simulink model "controller_dist_def_controller"  (R2018b)
settings: Solver=VariableStepAuto  StartTime=0.0  StopTime=30  MaxStep=1e-3  RelTol=1e-3
InitFcn:
  | % NOTE: If using VoltPAQ-X1, make sure both Gain switches are set to 3.
  | K_AMP = 3;
  | % Maximum Output Voltage (V): YAW limited to 15 V. PITCH limited to 24 V.
  | VMAX_AMP_P = 24;
  | VMAX_AMP_Y = 15;
  | % Initial Angle of Pitch (rad)
  | theta_0 = -40.5*pi/180;
  | 
  | g = 9.81;
  | 
  | % Pitch and Yaw Motor Armature Resistance (Ohm)
  | R_m_p = 0.83;
  | R_m_y = 1.60;
  | 
  | % Pitch and Yaw Motor Current-Torque Constant (N.m/A)
  | K_t_p = 0.0182;
  | K_t_y = 0.0109;
  | 
  | % Pitch and Yaw Motor Voltage-Torque Constant (N.m/V)
  | K_yp = K_t_p / R_m_p;
  | K_py = K_t_y / R_m_y;
  | 
  | % Pitch and Yaw Viscous Damping Constant (N.m.s/rad)
  | B_p = 0.8;  % tuned while running simulation and experiment in parallel
  | B_y = 0.318; % identified as described in manual
  | 
  | % Mass of the Helicopter (kg)
  | m_heli = 1.3872;
  | 
  | % Mass of the Helicopter with Yoke (kg)
  | m_heli_case = 1.421;
  | 
  | % Distance from Pitch Pivot to Pitch/Front Motor and Yaw/Back Motor(m)
  | r_p = 7.75*0.0254;
  | r_y = (6+5/8)*0.0254;
  | 
  | % Pitch and Yaw Propeller Force-Thrust Constant found Experimentally (N/V)
  | K_f_p = 5*0.2074;
  | K_f_y = 3*0.1426;
  | 
  | % Pitch and Yaw Propeller Torque-Thrust Constant found Experimentally (N.m/V)
  | K_pp = K_f_p * r_p;
  | K_yy = K_f_y * r_y;
  | 
  | % Mass of Pitch/Front Motor and Yaw/Back Motor (kg)
  | m_motor_p = 0.292;
  | m_motor_y = 0.128;
  | 
  | % Mass of Pitch/Front and Yaw/Back Guard + Propeller(kg)
  | m_shield = 0.143 + 0.024;
  | 
  | % Total Mass of Pitch and Yaw Motor/Shield Assemblies (kg)
  | m_props = ( m_motor_p + m_motor_y + 2 * m_shield );
  | 
  | % Mass of Helicopter Body moving about Pitch Axis (kg)
  | m_body_p = m_heli - m_props;
  | 
  | % Mass of Helicopter Body moving about Yaw Axis (kg)
  | m_body_y = m_heli_case - m_props;
  | 
  | % Mass of Metal Shaft Moving about Yaw Axis (kg)
  | m_shaft = 0.151;
  | 
  | % Total Length of Helicopter Body (m)
  | L_body = 19*0.0254;
  | 
  | % Helicopter Center of Mass from Pivot along Pitch Axis (m)
  | l_cm = ( (m_motor_p + m_shield ) * r_p +  (m_motor_y + m_shield ) * r_y ) / ( m_props ) ;
  | 
  | % Length of Metal Shaft Moving about Yaw Axis through slip ring (m)
  | L_shaft = 11 * 0.0254;
  | 
  | % Pitch and Yaw Motor Rotor Moment of Inertia (kg.m^2)
  | J_m_p = 1.91e-6; %1.7070e-5;
  | J_m_y = 1.374e-4; %1.4471e-5;
  | 
  | % Moment of Inertia of Helicopter Body about its CM (kg.m^2)
  | J_body_p = m_body_p * L_body^2 / 12;
  | J_body_y = m_body_y * L_body^2 / 12;
  | 
  | % Moment of Inertia of Metal Shaft about Yaw Axis (kg.m^2)
  | J_shaft = m_shaft * L_shaft^2 / 3; %;0.0851;
  | 
  | % Moment of Inertia of Pitch Motor + Guard Assembly about Pivot (kg.m^2)
  | J_p = ( m_motor_p + m_shield ) * r_p^2;
  | 
  | % Moment of Inertia of Yaw Motor + Guard Assembly about Pivot (kg.m^2)
  | J_y = ( m_motor_y + m_shield ) * r_y^2;
  | 
  | % Equivalent Moment of Inertia about Pitch and Yaw Axis (kg.m^2)
  | J_eq_p = J_m_p + J_body_p + J_p + J_y;
  | J_eq_y = J_m_y + J_body_y + J_p + J_y + J_shaft;
  | 
  | 
  | %BESSEL wn=4
  | Kbes=[     68.5119  -25.1203    5.3421   -3.6881
  |    63.1652  188.4894    0.7783   19.4789];
  | 
  | xd=-20;
settings Model: Creator=rezan  LastModifiedBy=rezan
settings DataIOCC: ReturnWorkspaceOutputs=on
settings DebuggingCC: UnconnectedInputMsg=none  UnconnectedOutputMsg=none  UnconnectedLineMsg=none  SFMachineParentedDataDiag=error

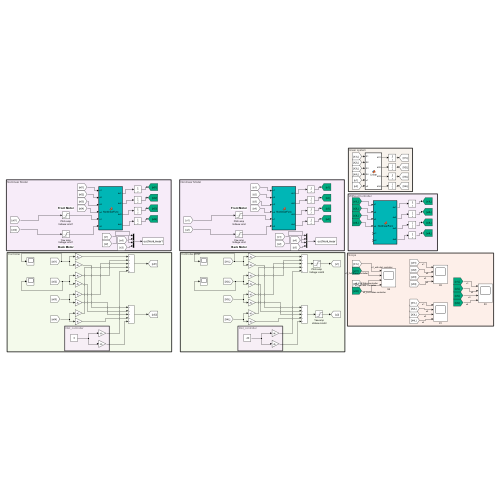
[thumbnail: Simulink's stored preview of the top-level diagram]
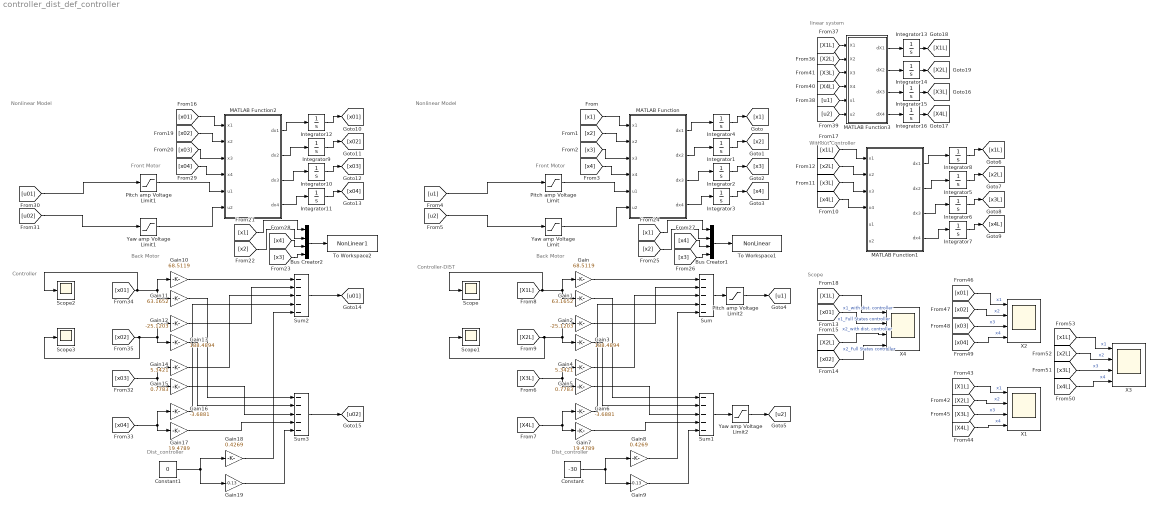
== system controller_dist_def_controller ==
  note: Dist_controller
  note: Controller-DIST
  note: Scope
  note: Nonlinear Model
  note: Front Motor
  note: Back Motor
  note: Without Controller
  note: Dist_controller
  note: Controller
  note: Nonlinear Model
  note: Front Motor
  note: Back Motor
  note: linear system
  Bus Creator1 : BusCreator  Inputs=4
  Bus Creator2 : BusCreator  Inputs=4
  Constant : Constant  Value=-30
  Constant1 : Constant  Value=0
  Gain : Gain  Gain=68.5119
  Gain1 : Gain  Gain=63.1652
  Gain10 : Gain  Gain=68.5119
  Gain11 : Gain  Gain=63.1652
  Gain12 : Gain  Gain=-25.1203
  Gain13 : Gain  Gain=188.4894
  Gain14 : Gain  Gain=5.3421
  Gain15 : Gain  Gain=0.7783
  Gain16 : Gain  Gain=-3.6881
  Gain17 : Gain  Gain=19.4789
  Gain18 : Gain  Gain=0.4269
  Gain19 : Gain  Gain=-0.13
  Gain2 : Gain  Gain=-25.1203
  Gain3 : Gain  Gain=188.4894
  Gain4 : Gain  Gain=5.3421
  Gain5 : Gain  Gain=0.7783
  Gain6 : Gain  Gain=-3.6881
  Gain7 : Gain  Gain=19.4789
  Gain8 : Gain  Gain=0.4269
  Gain9 : Gain  Gain=-0.13
  Integrator{1..3,5,7,9,11,14,16} (9 alike) : Integrator
  Integrator10 : Integrator  InitialCondition=5
  Integrator{4,8,12..13} (4 alike) : Integrator  UpperSaturationLimit=40.5*pi/180  LowerSaturationLimit=-40.5*pi/180
  Integrator15 : Integrator  InitialCondition=5
  Integrator6 : Integrator  InitialCondition=5
  MATLAB Function : MATLAB Function  TreatAsAtomicUnit=on
  MATLAB Function1 : MATLAB Function  TreatAsAtomicUnit=on
  MATLAB Function2 : MATLAB Function  TreatAsAtomicUnit=on
  MATLAB Function3 : MATLAB Function  TreatAsAtomicUnit=on
  Pitch amp Voltage Limit : Saturate  UpperLimit=VMAX_AMP_P  LowerLimit=- VMAX_AMP_P
  Pitch amp Voltage Limit1 : Saturate  UpperLimit=VMAX_AMP_P  LowerLimit=- VMAX_AMP_P
  Pitch amp Voltage Limit2 : Saturate  UpperLimit=VMAX_AMP_P  LowerLimit=- VMAX_AMP_P
  Scope{,1..3} (4 alike) : Scope
  Sum{,1..3} (4 alike) : Sum  Inputs=-----
  To Workspace1 : ToWorkspace  VariableName=NonLinear  SampleTime=-1
  To Workspace2 : ToWorkspace  VariableName=NonLinear1  SampleTime=-1
  X{1..4} (4 alike) : Scope  NumInputPorts=4
  Yaw amp Voltage Limit : Saturate  UpperLimit=VMAX_AMP_Y  LowerLimit=- VMAX_AMP_Y
  Yaw amp Voltage Limit1 : Saturate  UpperLimit=VMAX_AMP_Y  LowerLimit=- VMAX_AMP_Y
  Yaw amp Voltage Limit2 : Saturate  UpperLimit=VMAX_AMP_Y  LowerLimit=- VMAX_AMP_Y
  wires:
  [x4] -> MATLAB Function/4(x4)
  [x2] -> MATLAB Function/2(x2)
  Integrator1/1 -> [x2]
  [u1] -> Pitch amp Voltage Limit/1
  [x1] -> MATLAB Function/1(x1)
  [u2] -> Yaw amp Voltage Limit/1
  MATLAB Function/1(dx1) -> Integrator4/1
  MATLAB Function/3(dx3) -> Integrator2/1
  MATLAB Function/2(dx2) -> Integrator1/1
  [x2] -> Bus Creator1/2
  [x4] -> Bus Creator1/3
  [x3] -> Bus Creator1/4
  Bus Creator1/1 -> To Workspace1/1
  Yaw amp Voltage Limit/1 -> MATLAB Function/6(u2)
  [x1] -> Bus Creator1/1
  Integrator3/1 -> [x4]
  Integrator4/1 -> [x1]
  MATLAB Function/4(dx4) -> Integrator3/1
  [x3] -> MATLAB Function/3(x3)
  Integrator2/1 -> [x3]
  Pitch amp Voltage Limit/1 -> MATLAB Function/5(u1)
  [X1L] -> Scope/1, Gain1/1, Gain/1
  [X4L] -> Gain7/1, Gain6/1
  [X3L] -> Gain4/1, Gain5/1
  Gain/1 -> Sum/1
  Gain2/1 -> Sum/2
  Gain4/1 -> Sum/3
  Gain6/1 -> Sum/4
  Gain3/1 -> Sum1/2
  Gain1/1 -> Sum1/1
  Gain5/1 -> Sum1/3
  Gain7/1 -> Sum1/4
  Sum/1 -> Pitch amp Voltage Limit2/1
  Sum1/1 -> Yaw amp Voltage Limit2/1
  Constant/1 -> Gain9/1, Gain8/1
  Gain8/1 -> Sum/5
  Gain9/1 -> Sum1/5
  [X2L] -> Scope1/1, Gain2/1, Gain3/1
  Integrator6/1 -> [x3L]
  Integrator8/1 -> [x1L]
  MATLAB Function1/4(dx4) -> Integrator7/1
  Integrator7/1 -> [x4L]
  [x3L] -> MATLAB Function1/3(x3)
  [x1L] -> MATLAB Function1/1(x1)
  MATLAB Function1/1(dx1) -> Integrator8/1
  MATLAB Function1/2(dx2) -> Integrator5/1
  [x2L] -> MATLAB Function1/2(x2)
  Integrator5/1 -> [x2L]
  MATLAB Function1/3(dx3) -> Integrator6/1
  [x4L] -> MATLAB Function1/4(x4)
  [X1L] -> X4/1  "x1_with dist. controller"
  [x01] -> X4/2  "x1_Full States controller"
  [X2L] -> X4/3  "x2_with dist. controller"
  [x02] -> X4/4  "x2_Full States controller"
  [x02] -> Gain13/1, Gain12/1, Scope3/1
  Gain19/1 -> Sum3/5
  Gain18/1 -> Sum2/5
  Constant1/1 -> Gain18/1, Gain19/1
  Sum3/1 -> [u02]
  Sum2/1 -> [u01]
  Gain17/1 -> Sum3/4
  Gain15/1 -> Sum3/3
  Gain11/1 -> Sum3/1
  Gain13/1 -> Sum3/2
  Gain16/1 -> Sum2/4
  Gain14/1 -> Sum2/3
  Gain12/1 -> Sum2/2
  Gain10/1 -> Sum2/1
  [x03] -> Gain15/1, Gain14/1
  [x04] -> Gain16/1, Gain17/1
  [x01] -> Gain10/1, Gain11/1, Scope2/1
  Pitch amp Voltage Limit1/1 -> MATLAB Function2/5(u1)
  Integrator10/1 -> [x03]
  [x03] -> MATLAB Function2/3(x3)
  MATLAB Function2/4(dx4) -> Integrator11/1
  Integrator12/1 -> [x01]
  Integrator11/1 -> [x04]
  [x1] -> Bus Creator2/1
  Yaw amp Voltage Limit1/1 -> MATLAB Function2/6(u2)
  Bus Creator2/1 -> To Workspace2/1
  [x3] -> Bus Creator2/4
  [x4] -> Bus Creator2/3
  [x2] -> Bus Creator2/2
  MATLAB Function2/2(dx2) -> Integrator9/1
  MATLAB Function2/3(dx3) -> Integrator10/1
  MATLAB Function2/1(dx1) -> Integrator12/1
  [u02] -> Yaw amp Voltage Limit1/1
  [x01] -> MATLAB Function2/1(x1)
  [u01] -> Pitch amp Voltage Limit1/1
  Integrator9/1 -> [x02]
  [x02] -> MATLAB Function2/2(x2)
  [x04] -> MATLAB Function2/4(x4)
  Integrator15/1 -> [X3L]
  [X4L] -> MATLAB Function3/4(X4)
  [X3L] -> MATLAB Function3/3(X3)
  MATLAB Function3/3(dX3) -> Integrator15/1
  MATLAB Function3/1(dX1) -> Integrator13/1
  MATLAB Function3/4(dX4) -> Integrator16/1
  Integrator13/1 -> [X1L]
  Integrator16/1 -> [X4L]
  MATLAB Function3/2(dX2) -> Integrator14/1
  [u1] -> MATLAB Function3/5(u1)
  [u2] -> MATLAB Function3/6(u2)
  [X2L] -> MATLAB Function3/2(X2)
  Integrator14/1 -> [X2L]
  [X1L] -> MATLAB Function3/1(X1)
  Pitch amp Voltage Limit2/1 -> [u1]
  Yaw amp Voltage Limit2/1 -> [u2]
  [X1L] -> X1/1  "x1"
  [X2L] -> X1/2  "x2"
  [X3L] -> X1/3  "x3"
  [X4L] -> X1/4  "x4"
  [x01] -> X2/1  "x1"
  [x02] -> X2/2  "x2"
  [x03] -> X2/3  "x3"
  [x04] -> X2/4  "x4"
  [x4L] -> X3/4  "x4"
  [x3L] -> X3/3  "x3"
  [x2L] -> X3/2  "x2"
  [x1L] -> X3/1  "x1"

== matlab function controller_dist_def_controller/MATLAB Function1 ==
  data: x1 input; x2 input; x3 input; x4 input; u1 input; dx1 output; u2 input; dx2 output; dx3 output; dx4 output
function [dx1,dx2,dx3,dx4]= NonlinearFunc(x1,x2,x3,x4,u1,u2)
%% Initial Conditions
% Gravitational Constant (m/s^2)
g = 9.81;

% Pitch and Yaw Motor Armature Resistance (Ohm)
R_m_p = 0.83;
R_m_y = 1.60;

% Pitch and Yaw Motor Current-Torque Constant (N.m/A)
K_t_p = 0.0182;
K_t_y = 0.0109;

% Pitch and Yaw Motor Voltage-Torque Constant (N.m/V)
K_yp = K_t_p / R_m_p;
K_py = K_t_y / R_m_y;

% Pitch and Yaw Viscous Damping Constant (N.m.s/rad)
B_p = 0.8;  % tuned while running simulation and experiment in parallel
B_y = 0.318; % identified as described in manual 

% Mass of the Helicopter (kg)
m_heli = 1.3872;

% Mass of the Helicopter with Yoke (kg)
m_heli_case = 1.421;

% Distance from Pitch Pivot to Pitch/Front Motor and Yaw/Back Motor(m)
r_p = 7.75*0.0254;
r_y = (6+5/8)*0.0254;

% Pitch and Yaw Propeller Force-Thrust Constant found Experimentally (N/V)
K_f_p = 5*0.2074;
K_f_y = 3*0.1426;

% Pitch and Yaw Propeller Torque-Thrust Constant found Experimentally (N.m/V)
K_pp = K_f_p * r_p;
K_yy = K_f_y * r_y;

% Mass of Pitch/Front Motor and Yaw/Back Motor (kg)
m_motor_p = 0.292;
m_motor_y = 0.128;

% Mass of Pitch/Front and Yaw/Back Guard + Propeller(kg)
m_shield = 0.143 + 0.024;

% Total Mass of Pitch and Yaw Motor/Shield Assemblies (kg)
m_props = ( m_motor_p + m_motor_y + 2 * m_shield );

% Mass of Helicopter Body moving about Pitch Axis (kg)
m_body_p = m_heli - m_props; 

% Mass of Helicopter Body moving about Yaw Axis (kg)
m_body_y = m_heli_case - m_props; 

% Mass of Metal Shaft Moving about Yaw Axis (kg)
m_shaft = 0.151;

% Total Length of Helicopter Body (m)
L_body = 19*0.0254;

% Helicopter Center of Mass from Pivot along Pitch Axis (m)
l_cm = ( (m_motor_p + m_shield ) * r_p +  (m_motor_y + m_shield ) * r_y ) / ( m_props ) ;

% Length of Metal Shaft Moving about Yaw Axis through slip ring (m)
L_shaft = 11 * 0.0254;

% Pitch and Yaw Motor Rotor Moment of Inertia (kg.m^2)
J_m_p = 1.91e-6; %1.7070e-5;
J_m_y = 1.374e-4; %1.4471e-5;

% Moment of Inertia of Helicopter Body about its CM (kg.m^2)
J_body_p = m_body_p * L_body^2 / 12;
J_body_y = m_body_y * L_body^2 / 12;

% Moment of Inertia of Metal Shaft about Yaw Axis (kg.m^2)
J_shaft = m_shaft * L_shaft^2 / 3; %;0.0851;

% Moment of Inertia of Pitch Motor + Guard Assembly about Pivot (kg.m^2)
J_p = ( m_motor_p + m_shield ) * r_p^2;

% Moment of Inertia of Yaw Motor + Guard Assembly about Pivot (kg.m^2)
J_y = ( m_motor_y + m_shield ) * r_y^2;

% Equivalent Moment of Inertia about Pitch and Yaw Axis (kg.m^2)
J_eq_p = J_m_p + J_body_p + J_p + J_y;
J_eq_y = J_m_y + J_body_y + J_p + J_y + J_shaft;
%%
%%
xd=-30;
 dx1=x3;
dx2=x4;
dx3=(1/(J_eq_p +m_heli*l_cm^2))*((K_pp*u1+K_py*u2)-(B_p*x3+m_heli*l_cm^2*x4^2*sin(x1)*cos(x1)+m_heli*g*l_cm*cos(x1)));
dx3=dx3+xd;
dx4=1/(J_eq_y + m_heli *l_cm^2* (cos(x1))^2 )*((K_yp*u1 )+(K_yy*u2 ))+(-B_y*x4+2*m_heli*l_cm^2*x4*x3*sin(x1)*cos(x1))/(J_eq_p+ m_heli * l_cm^2 * (cos(x1))^2);

== matlab function controller_dist_def_controller/MATLAB Function2 ==
  data: x1 input; x2 input; x3 input; x4 input; u1 input; dx1 output; u2 input; dx2 output; dx3 output; dx4 output
function [dx1,dx2,dx3,dx4]= NonlinearFunc(x1,x2,x3,x4,u1,u2)
%% Initial Conditions
% Gravitational Constant (m/s^2)
g = 9.81;

% Pitch and Yaw Motor Armature Resistance (Ohm)
R_m_p = 0.83;
R_m_y = 1.60;

% Pitch and Yaw Motor Current-Torque Constant (N.m/A)
K_t_p = 0.0182;
K_t_y = 0.0109;

% Pitch and Yaw Motor Voltage-Torque Constant (N.m/V)
K_yp = K_t_p / R_m_p;
K_py = K_t_y / R_m_y;

% Pitch and Yaw Viscous Damping Constant (N.m.s/rad)
B_p = 0.8;  % tuned while running simulation and experiment in parallel
B_y = 0.318; % identified as described in manual 

% Mass of the Helicopter (kg)
m_heli = 1.3872;

% Mass of the Helicopter with Yoke (kg)
m_heli_case = 1.421;

% Distance from Pitch Pivot to Pitch/Front Motor and Yaw/Back Motor(m)
r_p = 7.75*0.0254;
r_y = (6+5/8)*0.0254;

% Pitch and Yaw Propeller Force-Thrust Constant found Experimentally (N/V)
K_f_p = 5*0.2074;
K_f_y = 3*0.1426;

% Pitch and Yaw Propeller Torque-Thrust Constant found Experimentally (N.m/V)
K_pp = K_f_p * r_p;
K_yy = K_f_y * r_y;

% Mass of Pitch/Front Motor and Yaw/Back Motor (kg)
m_motor_p = 0.292;
m_motor_y = 0.128;

% Mass of Pitch/Front and Yaw/Back Guard + Propeller(kg)
m_shield = 0.143 + 0.024;

% Total Mass of Pitch and Yaw Motor/Shield Assemblies (kg)
m_props = ( m_motor_p + m_motor_y + 2 * m_shield );

% Mass of Helicopter Body moving about Pitch Axis (kg)
m_body_p = m_heli - m_props; 

% Mass of Helicopter Body moving about Yaw Axis (kg)
m_body_y = m_heli_case - m_props; 

% Mass of Metal Shaft Moving about Yaw Axis (kg)
m_shaft = 0.151;

% Total Length of Helicopter Body (m)
L_body = 19*0.0254;

% Helicopter Center of Mass from Pivot along Pitch Axis (m)
l_cm = ( (m_motor_p + m_shield ) * r_p +  (m_motor_y + m_shield ) * r_y ) / ( m_props ) ;

% Length of Metal Shaft Moving about Yaw Axis through slip ring (m)
L_shaft = 11 * 0.0254;

% Pitch and Yaw Motor Rotor Moment of Inertia (kg.m^2)
J_m_p = 1.91e-6; %1.7070e-5;
J_m_y = 1.374e-4; %1.4471e-5;

% Moment of Inertia of Helicopter Body about its CM (kg.m^2)
J_body_p = m_body_p * L_body^2 / 12;
J_body_y = m_body_y * L_body^2 / 12;

% Moment of Inertia of Metal Shaft about Yaw Axis (kg.m^2)
J_shaft = m_shaft * L_shaft^2 / 3; %;0.0851;

% Moment of Inertia of Pitch Motor + Guard Assembly about Pivot (kg.m^2)
J_p = ( m_motor_p + m_shield ) * r_p^2;

% Moment of Inertia of Yaw Motor + Guard Assembly about Pivot (kg.m^2)
J_y = ( m_motor_y + m_shield ) * r_y^2;

% Equivalent Moment of Inertia about Pitch and Yaw Axis (kg.m^2)
J_eq_p = J_m_p + J_body_p + J_p + J_y;
J_eq_y = J_m_y + J_body_y + J_p + J_y + J_shaft;
%%
%%
xd=-30
 dx1=x3;
dx2=x4;
dx3=(1/(J_eq_p +m_heli*l_cm^2))*((K_pp*u1+K_py*u2)-(B_p*x3+m_heli*l_cm^2*x4^2*sin(x1)*cos(x1)+m_heli*g*l_cm*cos(x1)));
dx3=dx3+xd;
dx4=1/(J_eq_y + m_heli *l_cm^2* (cos(x1))^2 )*((K_yp*u1 )+(K_yy*u2 ))+(-B_y*x4+2*m_heli*l_cm^2*x4*x3*sin(x1)*cos(x1))/(J_eq_p+ m_heli * l_cm^2 * (cos(x1))^2);

== matlab function controller_dist_def_controller/MATLAB Function3 ==
  data: X1 input; dX1 output; X2 input; X3 input; X4 input; u1 input; dX2 output; dX3 output; dX4 output; u2 input
function [dX1,dX2,dX3,dX4] = Linear(X1,X2,X3,X4,u1,u2)
%#codegen

A=[      0         0    1.0000         0
         0         0         0    1.0000
         0         0   -9.2751         0
         0         0         0   -3.4955];
     
B=[      0         0
         0         0
    2.3667    0.0790
    0.2410    0.7913];

X = [X1;X2;X3;X4];
U=[u1,u2].';
dX = A*X+B*U;
xd=-30;

dX1 = dX(1);
dX2 = dX(2);
dX3 = dX(3)+xd;
dX4 = dX(4);

== matlab function controller_dist_def_controller/MATLAB Function ==
  data: x1 input; x2 input; x3 input; x4 input; u1 input; dx1 output; u2 input; dx2 output; dx3 output; dx4 output
function [dx1,dx2,dx3,dx4]= NonlinearFunc(x1,x2,x3,x4,u1,u2)
%% Initial Conditions
% Gravitational Constant (m/s^2)
g = 9.81;

% Pitch and Yaw Motor Armature Resistance (Ohm)
R_m_p = 0.83;
R_m_y = 1.60;

% Pitch and Yaw Motor Current-Torque Constant (N.m/A)
K_t_p = 0.0182;
K_t_y = 0.0109;

% Pitch and Yaw Motor Voltage-Torque Constant (N.m/V)
K_yp = K_t_p / R_m_p;
K_py = K_t_y / R_m_y;

% Pitch and Yaw Viscous Damping Constant (N.m.s/rad)
B_p = 0.8;  % tuned while running simulation and experiment in parallel
B_y = 0.318; % identified as described in manual 

% Mass of the Helicopter (kg)
m_heli = 1.3872;

% Mass of the Helicopter with Yoke (kg)
m_heli_case = 1.421;

% Distance from Pitch Pivot to Pitch/Front Motor and Yaw/Back Motor(m)
r_p = 7.75*0.0254;
r_y = (6+5/8)*0.0254;

% Pitch and Yaw Propeller Force-Thrust Constant found Experimentally (N/V)
K_f_p = 5*0.2074;
K_f_y = 3*0.1426;

% Pitch and Yaw Propeller Torque-Thrust Constant found Experimentally (N.m/V)
K_pp = K_f_p * r_p;
K_yy = K_f_y * r_y;

% Mass of Pitch/Front Motor and Yaw/Back Motor (kg)
m_motor_p = 0.292;
m_motor_y = 0.128;

% Mass of Pitch/Front and Yaw/Back Guard + Propeller(kg)
m_shield = 0.143 + 0.024;

% Total Mass of Pitch and Yaw Motor/Shield Assemblies (kg)
m_props = ( m_motor_p + m_motor_y + 2 * m_shield );

% Mass of Helicopter Body moving about Pitch Axis (kg)
m_body_p = m_heli - m_props; 

% Mass of Helicopter Body moving about Yaw Axis (kg)
m_body_y = m_heli_case - m_props; 

% Mass of Metal Shaft Moving about Yaw Axis (kg)
m_shaft = 0.151;

% Total Length of Helicopter Body (m)
L_body = 19*0.0254;

% Helicopter Center of Mass from Pivot along Pitch Axis (m)
l_cm = ( (m_motor_p + m_shield ) * r_p +  (m_motor_y + m_shield ) * r_y ) / ( m_props ) ;

% Length of Metal Shaft Moving about Yaw Axis through slip ring (m)
L_shaft = 11 * 0.0254;

% Pitch and Yaw Motor Rotor Moment of Inertia (kg.m^2)
J_m_p = 1.91e-6; %1.7070e-5;
J_m_y = 1.374e-4; %1.4471e-5;

% Moment of Inertia of Helicopter Body about its CM (kg.m^2)
J_body_p = m_body_p * L_body^2 / 12;
J_body_y = m_body_y * L_body^2 / 12;

% Moment of Inertia of Metal Shaft about Yaw Axis (kg.m^2)
J_shaft = m_shaft * L_shaft^2 / 3; %;0.0851;

% Moment of Inertia of Pitch Motor + Guard Assembly about Pivot (kg.m^2)
J_p = ( m_motor_p + m_shield ) * r_p^2;

% Moment of Inertia of Yaw Motor + Guard Assembly about Pivot (kg.m^2)
J_y = ( m_motor_y + m_shield ) * r_y^2;

% Equivalent Moment of Inertia about Pitch and Yaw Axis (kg.m^2)
J_eq_p = J_m_p + J_body_p + J_p + J_y;
J_eq_y = J_m_y + J_body_y + J_p + J_y + J_shaft;
%%
%%
xd=-30
 dx1=x3;
dx2=x4;
dx3=(1/(J_eq_p +m_heli*l_cm^2))*((K_pp*u1+K_py*u2)-(B_p*x3+m_heli*l_cm^2*x4^2*sin(x1)*cos(x1)+m_heli*g*l_cm*cos(x1)));
dx3=dx3+xd;
dx4=1/(J_eq_y + m_heli *l_cm^2* (cos(x1))^2 )*((K_yp*u1 )+(K_yy*u2 ))+(-B_y*x4+2*m_heli*l_cm^2*x4*x3*sin(x1)*cos(x1))/(J_eq_p+ m_heli * l_cm^2 * (cos(x1))^2);
